simulink model "CubeSatSimulationModel"  (R2024b)
settings: Solver=VariableStepAuto  StartTime=0.0  StopTime=500  MaxStep=0.2  RelTol=1e-3
undefined symbols (not defined in the file or in its folder): IAU, juliandate, mtq, sat, WMM2020
libraries: matrix_library x10, aerolibutil x9, sharedutil x4, aerolibgravity2 x2, simulink_extras x2, sharedtransform x2, aerolibtransform2 x1, simulink x1
settings Model: PacingRate=3  Creator=Ameya  LastModifiedBy=Ameya
settings SFSimCC: SFSimEcho=off
settings RTWCC: GPUComputeCapability=3.5

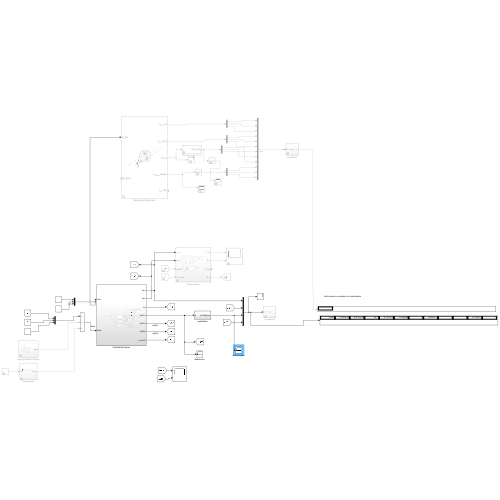
[thumbnail: Simulink's stored preview of the top-level diagram]
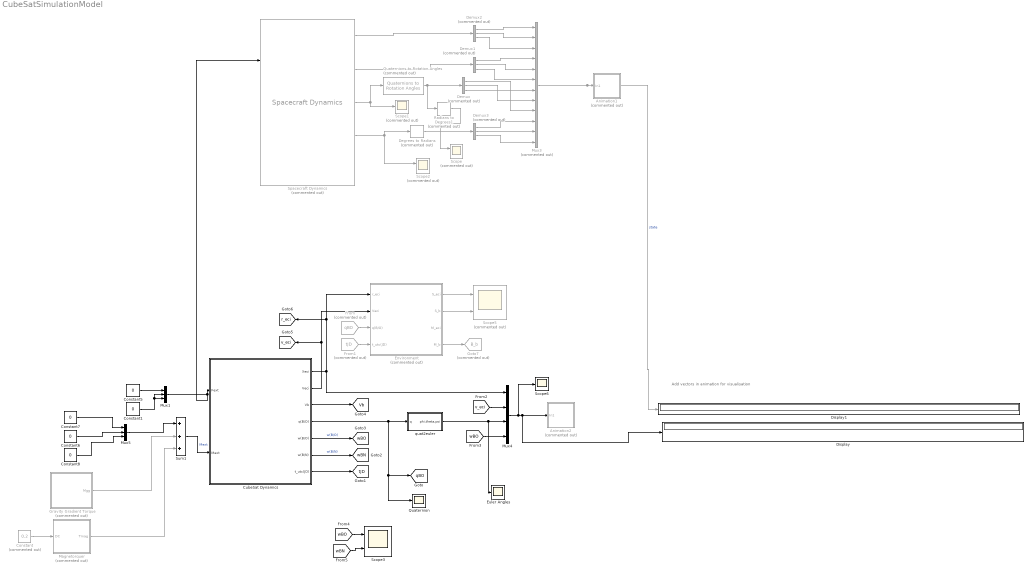
== system CubeSatSimulationModel ==
  note: Add vectors in animation for visualisation
  Animation1 : Subsystem  Commented=on
  Animation2 : Subsystem  Commented=on
  Constant : Constant  Commented=on  Value=0.2
  Constant{1,5..8} (5 alike) : Constant  Value=0
  CubeSat Dynamics : Subsystem
  Degrees to Radians : simulink_extras/Transformations/Degrees to Radians  Commented=on
  Demux{,1..3} (4 alike) : Demux  Commented=on  Outputs=3
  Display : Display
  Display1 : Display
  Environment : Subsystem  Commented=on
  Euler Angles : Scope
  From : From  Commented=on  GotoTag=qBO  TagVisibility=global
  From1 : From  Commented=on  GotoTag=tJD  TagVisibility=global
  Goto7 : Goto  Commented=on  GotoTag=B_b  TagVisibility=global
  Gravity Gradient Torque : Subsystem  Commented=on
  Magnetorquer : Subsystem  Commented=on
  Mux1 : Mux  Inputs=3
  Mux3 : Mux  Commented=on  Inputs=12
  Mux4 : Mux
  Mux5 : Mux  Inputs=3
  Quaternion : Scope
  Quaternions to Rotation Angles : sharedtransform/Quaternions to Rotation Angles  Commented=on  rotationOrder=ZYX  aMode=aMode
  Radians to Degrees1 : simulink_extras/Transformations/Radians to Degrees  Commented=on
  Scope : Scope  Commented=on  NumInputPorts=2
  Scope1 : Scope  Commented=on
  Scope2 : Scope  Commented=on  NumInputPorts=2
  Scope3 : Scope  NumInputPorts=2
  Scope5 : Scope  Commented=on  NumInputPorts=2
  Scope6 : Scope
  Spacecraft Dynamics : SpacecraftDynamics  Commented=on  mass=sat.mass  inertia=sat.J  semiMajorAxis=sat.a  eccentricity=sat.e  inclination=rad2deg(sat.i)  raan=rad2deg(sat.RAAN)  argPeriapsis=rad2deg(sat.w)  trueAnomaly=0  attitudeFrame=LVLH  attitudeRate=rad2deg(sat.w0)
  Sum1 : Sum  Inputs=+++
  quat2euler : Subsystem
  tag scope: Vb=global, qBO=global, r_eci=global, tJD=global, v_eci=global, wBN=global, wBO=global
  wires:
  Spacecraft Dynamics/3 -> Scope1/1, Quaternions to Rotation Angles/1
  Quaternions to Rotation Angles/1 -> Demux/1, Radians to Degrees1/1
  Mux1/1 -> Spacecraft Dynamics/1, CubeSat Dynamics/1(Fext)
  Constant1/1 -> Mux1/2, Mux1/3
  Mux3/1 -> Animation1/1(In1), Display1/1  "state"
  Spacecraft Dynamics/2 -> Demux1/1
  Spacecraft Dynamics/1 -> Demux2/1
  Demux2/1 -> Mux3/1
  Demux2/2 -> Mux3/2
  Demux2/3 -> Mux3/3
  Demux1/1 -> Mux3/4
  Demux1/2 -> Mux3/5
  Demux1/3 -> Mux3/6
  Demux/1 -> Mux3/9
  Demux/2 -> Mux3/8
  Demux/3 -> Mux3/7
  Spacecraft Dynamics/4 -> Scope2/1, Degrees to Radians/1
  Demux3/1 -> Mux3/10
  Demux3/2 -> Mux3/11
  Demux3/3 -> Mux3/12
  Degrees to Radians/1 -> Demux3/1
  Radians to Degrees1/1 -> Scope/1
  CubeSat Dynamics/3(Vb) -> [Vb]
  Mux4/1 -> Scope6/1, Display/1, Animation2/1(In1)
  Constant5/1 -> Mux1/1
  quat2euler/1(phi,theta,psi) -> Mux4/3, Euler Angles/1
  CubeSat Dynamics/6(w(B/N)) -> [wBN]  "w(B/N)"
  CubeSat Dynamics/4(q(B/O)) -> [qBO], Quaternion/1, quat2euler/1(q)
  CubeSat Dynamics/1(Xeci) -> Environment/1(r_eci), [r_eci], Mux4/1
  From1/1 -> Environment/4(t_utc(JD))
  Environment/2(S_b) -> Scope5/2
  CubeSat Dynamics/2(Veci) -> [v_eci], Environment/2(Veci)
  From/1 -> Environment/3(q(B/O))
  CubeSat Dynamics/7(t_utc(JD)) -> [tJD]
  Environment/1(S_eci) -> Scope5/1
  Gravity Gradient Torque/1(Mgg) -> Sum1/2
  Mux5/1 -> Sum1/1
  Constant6/1 -> Mux5/2
  Sum1/1 -> CubeSat Dynamics/2(Mext)  "Mext"
  Constant8/1 -> Mux5/3
  Constant7/1 -> Mux5/1
  CubeSat Dynamics/5(w(B/O)) -> [wBO]  "w(B/O)"
  [v_eci] -> Mux4/2
  [wBO] -> Mux4/4
  Environment/4(M_b) -> Goto7/1
  Magnetorquer/1(Tmag) -> Sum1/3
  Constant/1 -> Magnetorquer/1(DC)
  [wBO] -> Scope3/1
  [wBN] -> Scope3/2

== system CubeSatSimulationModel/Animation1 ==
  In1 : Inport
  Clock : Clock
  CubeSat Attitude Animation : MATLABFcn  MATLABFcn=drawCubeSat  OutputDimensions=0
  Mux1 : Mux  Inputs=2
  wires:
  Mux1/1 -> CubeSat Attitude Animation/1
  In1/1 -> Mux1/1
  Clock/1 -> Mux1/2  "time"

== system CubeSatSimulationModel/Animation2 ==
  In1 : Inport
  Clock : Clock
  CubeSat Attitude Animation : MATLABFcn  MATLABFcn=drawCubeSat  OutputDimensions=0
  Mux1 : Mux  Inputs=2
  wires:
  Mux1/1 -> CubeSat Attitude Animation/1
  In1/1 -> Mux1/1
  Clock/1 -> Mux1/2  "time"

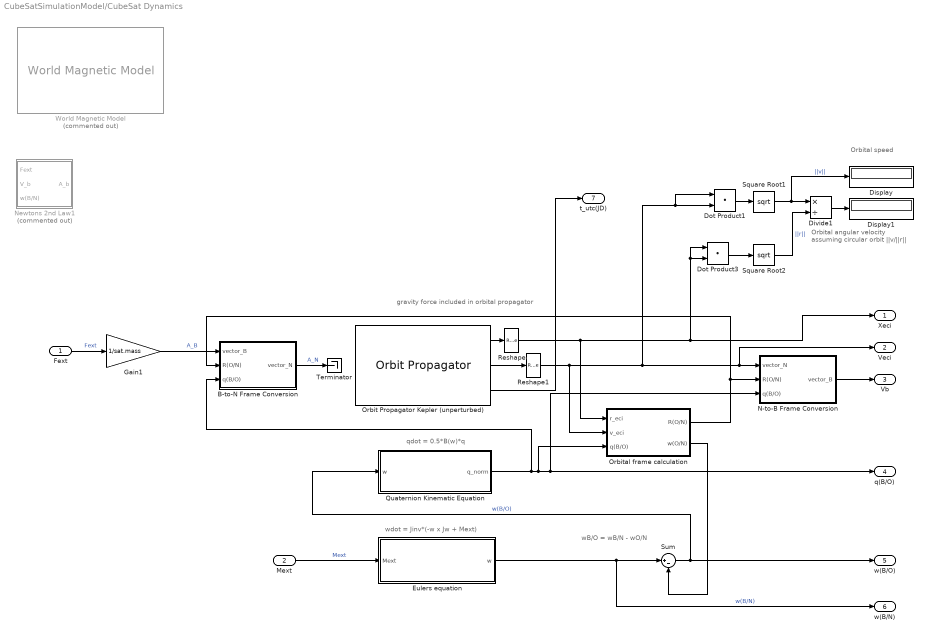
== system CubeSatSimulationModel/CubeSat Dynamics ==
  note: Orbital speed
  note: gravity force included in orbital propagator
  note: Orbital angular velocity
      | assuming circular orbit
      | ||v/||r||
  note: qdot = 0.5*B(w)*q
  note: wdot = Jinv*(-w x Jw + Mext)
  note: wB/O = wB/N - wO/N
  Fext : Inport
  Mext : Inport  Port=2
  B-to-N Frame Conversion : Subsystem
  Display : Display
  Display1 : Display
  Divide1 : Product  Inputs=*/
  Dot Product1 : DotProduct  OutDataTypeStr=Inherit: Inherit via internal rule
  Dot Product3 : DotProduct  OutDataTypeStr=Inherit: Inherit via internal rule
  Eulers equation : Subsystem
  Gain1 : Gain  Gain=1/sat.mass
  N-to-B Frame Conversion : Subsystem
  Newtons 2nd Law1 : Subsystem  Commented=on
  Orbit Propagator Kepler (unperturbed) : OrbitPropagator  accelIn=on  startDate=juliandate(2025, 1, 1, 12, 0, 0)  semiMajorAxis=sat.a  eccentricity=sat.e  inclination=rad2deg(sat.i)  raan=rad2deg(sat.RAAN)  argPeriapsis=rad2deg(sat.w)  trueAnomaly=rad2deg(sat.ta)  inertialPosition=[3649700.0 3308200.0 -4676600.0]  inertialVelocity=[-2750.8 6666.4 2573.4]  fixedPosition=[-4142689.0 -2676864.7 -4669861.6]  fixedVelocity=[1452.7 -6720.7 2568.1]  gravityModel=Oblate ellipsoid (J2)  customR=3396200  customMu=4.305e13  customJ2=1.0826269e-03  customOmega=4.06125949e-3
  Orbital frame calculation : Subsystem
  Quaternion Kinematic Equation : Subsystem
  Reshape : Reshape  OutputDimensionality=Column vector (2-D)
  Reshape1 : Reshape  OutputDimensionality=Column vector (2-D)
  Square Root1 : Sqrt
  Square Root2 : Sqrt
  Sum : Sum  Inputs=|+-
  Terminator : Terminator
  World Magnetic Model : aerolibgravity2/World Magnetic Model  Commented=on  model=WMM2020 (2020-2025)  customFile='WMM2020.COF'  units=Metric (MKS)  time_in=on  month=January  day=1  year=2020  action=Error  h_out=on  dec_out=on  inc_out=on  ti_out=on
  Xeci : Outport
  Veci : Outport  Port=2
  Vb : Outport  Port=3
  q(B/O) : Outport  Port=4
  w(B/O) : Outport  Port=5
  w(B/N) : Outport  Port=6
  t_utc(JD) : Outport  Port=7
  wires:
  Orbit Propagator Kepler (unperturbed)/1 -> Reshape/1
  Orbit Propagator Kepler (unperturbed)/2 -> Reshape1/1
  Reshape1/1 -> Dot Product1/1, Dot Product1/2, Veci/1, N-to-B Frame Conversion/1(vector_N), Orbital frame calculation/2(v_eci)
  Mext/1 -> Eulers equation/1(Mext)  "Mext"
  Eulers equation/1(w) -> w(B/N)/1, Sum/1  "w(B/N)"
  Sum/1 -> Quaternion Kinematic Equation/1(w), w(B/O)/1  "w(B/O)"
  Dot Product1/1 -> Square Root1/1
  Square Root1/1 -> Display/1, Divide1/1  "||v||"
  Dot Product3/1 -> Square Root2/1
  Square Root2/1 -> Divide1/2  "||r||"
  Divide1/1 -> Display1/1
  Quaternion Kinematic Equation/1(q_norm) -> q(B/O)/1, N-to-B Frame Conversion/3(q(B/O)), Orbital frame calculation/3(q(B/O)), B-to-N Frame Conversion/3(q(B/O))
  Orbital frame calculation/2(w(O/N)) -> Sum/2
  Reshape/1 -> Dot Product3/1, Dot Product3/2, Xeci/1, Orbital frame calculation/1(r_eci)
  Orbital frame calculation/1(R(O/N)) -> N-to-B Frame Conversion/2(R(O/N)), B-to-N Frame Conversion/2(R(O/N))
  Fext/1 -> Gain1/1  "Fext"
  N-to-B Frame Conversion/1(vector_B) -> Vb/1
  Gain1/1 -> B-to-N Frame Conversion/1(vector_B)  "A_B"
  B-to-N Frame Conversion/1(vector_N) -> Terminator/1  "A_N"
  Orbit Propagator Kepler (unperturbed)/3 -> t_utc(JD)/1

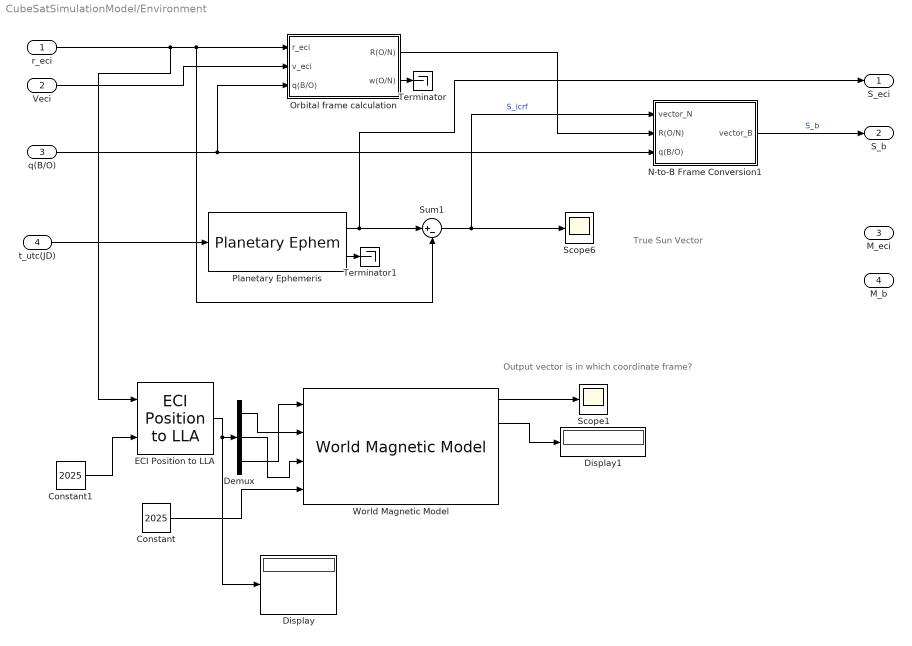
== system CubeSatSimulationModel/Environment ==
  note: Output vector is in which coordinate frame?
  note: True Sun Vector
  r_eci : Inport
  Veci : Inport  Port=2
  q(B/O) : Inport  Port=3
  t_utc(JD) : Inport  Port=4
  Constant : Constant  Value=2025
  Constant1 : Constant  Value=2025
  Demux : Demux  Outputs=3
  Display : Display
  Display1 : Display
  ECI Position to LLA : aerolibtransform2/ECI Position to LLA  red=IAU-2000/2006  year=2025  month=January  day=1  hour=0  min=0  sec=0  deltaT=Day  errorflag=Error  extraparamflag=off  eunits=Metric (MKS)  earthmodel=WGS84  flat=1/298.257223563  eqradius=6378137
      settings: AttributesFormatString=%<red>
  N-to-B Frame Conversion1 : Subsystem
  Orbital frame calculation : Subsystem
  Planetary Ephemeris : PlanetaryEphem  target=Sun
  Scope1 : Scope
  Scope6 : Scope
  Sum1 : Sum  Inputs=|+-
  Terminator : Terminator
  Terminator1 : Terminator
  World Magnetic Model : aerolibgravity2/World Magnetic Model  model=WMM2020 (2020-2025)  customFile='WMM2020.COF'  units=Metric (MKS)  time_in=on  month=January  day=1  year=2020  action=Error  h_out=on  dec_out=on  inc_out=on  ti_out=on
  S_eci : Outport
  S_b : Outport  Port=2
  M_eci : Outport  Port=3
  M_b : Outport  Port=4
  wires:
  Orbital frame calculation/1(R(O/N)) -> N-to-B Frame Conversion1/2(R(O/N))
  Sum1/1 -> Scope6/1, N-to-B Frame Conversion1/1(vector_N)  "S_icrf"
  Planetary Ephemeris/1 -> Sum1/1, S_eci/1
  q(B/O)/1 -> N-to-B Frame Conversion1/3(q(B/O)), Orbital frame calculation/3(q(B/O))
  r_eci/1 -> ECI Position to LLA/1, Orbital frame calculation/1(r_eci), Sum1/2
  t_utc(JD)/1 -> Planetary Ephemeris/1
  N-to-B Frame Conversion1/1(vector_B) -> S_b/1  "S_b"
  Planetary Ephemeris/2 -> Terminator1/1
  Orbital frame calculation/2(w(O/N)) -> Terminator/1
  Veci/1 -> Orbital frame calculation/2(v_eci)
  Demux/3 -> World Magnetic Model/1
  Demux/1 -> World Magnetic Model/2
  Demux/2 -> World Magnetic Model/3
  World Magnetic Model/1 -> Scope1/1
  Constant1/1 -> ECI Position to LLA/2
  Constant/1 -> World Magnetic Model/4
  ECI Position to LLA/1 -> Display/1, Demux/1
  World Magnetic Model/2 -> Display1/1

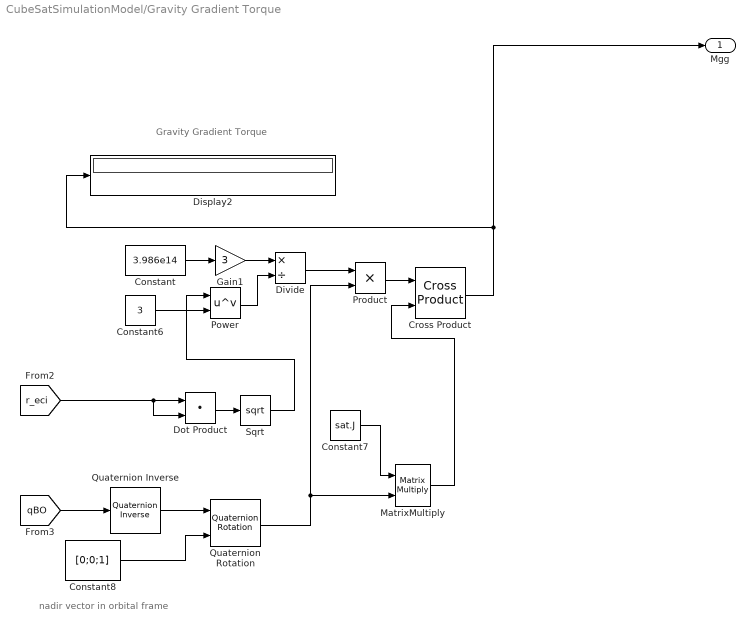
== system CubeSatSimulationModel/Gravity Gradient Torque ==
  note: Gravity Gradient Torque
  note: nadir vector in orbital frame
  Constant : Constant  Value=3.986e14
  Constant6 : Constant  Value=3
  Constant7 : Constant  Value=sat.J
  Constant8 : Constant  Value=[0;0;1]
  Cross Product : matrix_library/Cross Product
  Display2 : Display
  Divide : Product  Inputs=*/
  Dot Product : DotProduct  OutDataTypeStr=Inherit: Inherit via internal rule
  Gain1 : Gain  Gain=3
  MatrixMultiply : Product  Multiplication=Matrix(*)
  Power : Math  Operator=pow
  Product : Product
  Quaternion Inverse : aerolibutil/Quaternion Inverse
  Quaternion Rotation : aerolibutil/Quaternion Rotation
  Sqrt : Sqrt
  Mgg : Outport
  wires:
  Power/1 -> Divide/2
  Cross Product/1 -> Mgg/1, Display2/1
  MatrixMultiply/1 -> Cross Product/2
  Quaternion Inverse/1 -> Quaternion Rotation/1
  [qBO] -> Quaternion Inverse/1
  Sqrt/1 -> Power/1
  [r_eci] -> Dot Product/2, Dot Product/1
  Product/1 -> Cross Product/1
  Constant6/1 -> Power/2
  Dot Product/1 -> Sqrt/1
  Divide/1 -> Product/1
  Quaternion Rotation/1 -> Product/2, MatrixMultiply/2
  Gain1/1 -> Divide/1
  Constant/1 -> Gain1/1
  Constant8/1 -> Quaternion Rotation/2
  Constant7/1 -> MatrixMultiply/1

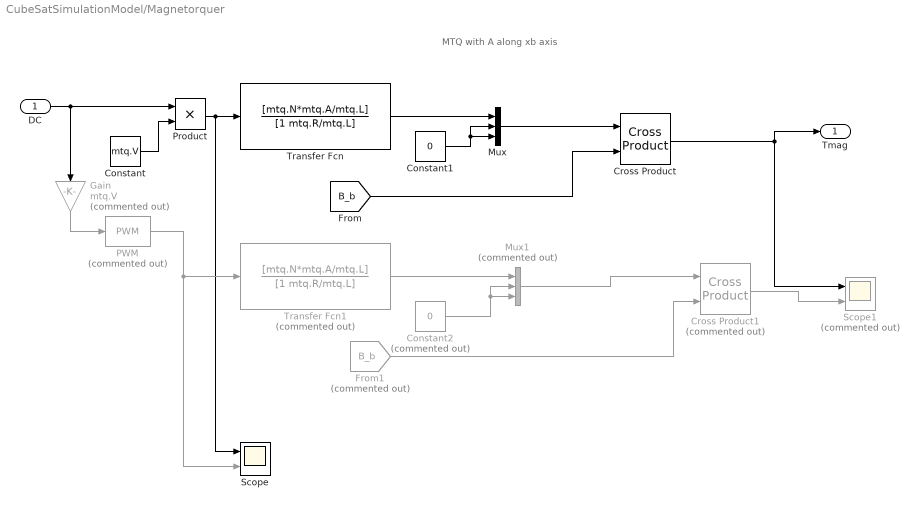
== system CubeSatSimulationModel/Magnetorquer ==
  note: MTQ with A along xb axis
  DC : Inport
  Constant : Constant  Value=mtq.V
  Constant1 : Constant  Value=0
  Constant2 : Constant  Commented=on  Value=0
  Cross Product : matrix_library/Cross Product
  Cross Product1 : matrix_library/Cross Product  Commented=on
  From1 : From  Commented=on  GotoTag=B_b  TagVisibility=global
  Gain : Gain  Commented=on  Gain=mtq.V
  Mux : Mux  Inputs=3
  Mux1 : Mux  Commented=on  Inputs=3
  PWM : simulink/Discontinuities/PWM  Commented=on  DisableCoverage=on  Period=1/50  InitialDelay=0  DisallowZeroDutyCycle=off  RunAtFixedTimeIntervals=off  SampleTime=0.1
  Product : Product
  Scope : Scope  NumInputPorts=2
  Scope1 : Scope  Commented=on  NumInputPorts=2
  Transfer Fcn : TransferFcn  Numerator=[mtq.N*mtq.A/mtq.L]  Denominator=[1 mtq.R/mtq.L]
  Transfer Fcn1 : TransferFcn  Commented=on  Numerator=[mtq.N*mtq.A/mtq.L]  Denominator=[1 mtq.R/mtq.L]
  Tmag : Outport
  wires:
  DC/1 -> Gain/1, Product/1
  Product/1 -> Scope/1, Transfer Fcn/1
  Constant/1 -> Product/2
  Transfer Fcn/1 -> Mux/1
  Cross Product/1 -> Tmag/1, Scope1/1
  [B_b] -> Cross Product/2
  PWM/1 -> Transfer Fcn1/1, Scope/2
  From1/1 -> Cross Product1/2
  Transfer Fcn1/1 -> Mux1/1
  Cross Product1/1 -> Scope1/2
  Constant1/1 -> Mux/2, Mux/3
  Mux/1 -> Cross Product/1
  Constant2/1 -> Mux1/2, Mux1/3
  Mux1/1 -> Cross Product1/1
  Gain/1 -> PWM/1

== system CubeSatSimulationModel/quat2euler ==
  q : Inport
  Demux4 : Demux  Outputs=3
  Mux5 : Mux  Inputs=3
  Quaternions to Rotation Angles1 : sharedtransform/Quaternions to Rotation Angles  rotationOrder=ZYX  aMode=aMode
  phi,theta,psi : Outport
  wires:
  Quaternions to Rotation Angles1/1 -> Demux4/1
  Demux4/3 -> Mux5/1
  Demux4/2 -> Mux5/2
  Demux4/1 -> Mux5/3
  q/1 -> Quaternions to Rotation Angles1/1
  Mux5/1 -> phi,theta,psi/1

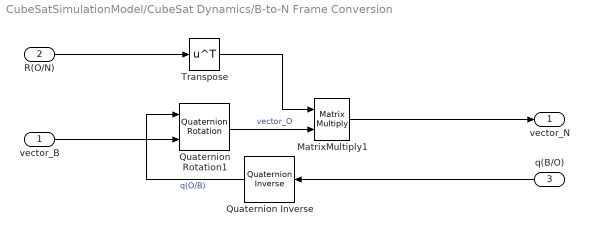
== system CubeSatSimulationModel/CubeSat Dynamics/B-to-N Frame Conversion ==
  vector_B : Inport
  R(O/N) : Inport  Port=2
  q(B/O) : Inport  Port=3
  MatrixMultiply1 : Product  Multiplication=Matrix(*)
  Quaternion Inverse : aerolibutil/Quaternion Inverse
  Quaternion Rotation1 : aerolibutil/Quaternion Rotation
  Transpose : Math  Operator=transpose
  vector_N : Outport
  wires:
  Transpose/1 -> MatrixMultiply1/1
  MatrixMultiply1/1 -> vector_N/1
  R(O/N)/1 -> Transpose/1
  Quaternion Inverse/1 -> Quaternion Rotation1/1  "q(O/B)"
  Quaternion Rotation1/1 -> MatrixMultiply1/2  "vector_O"
  q(B/O)/1 -> Quaternion Inverse/1
  vector_B/1 -> Quaternion Rotation1/2

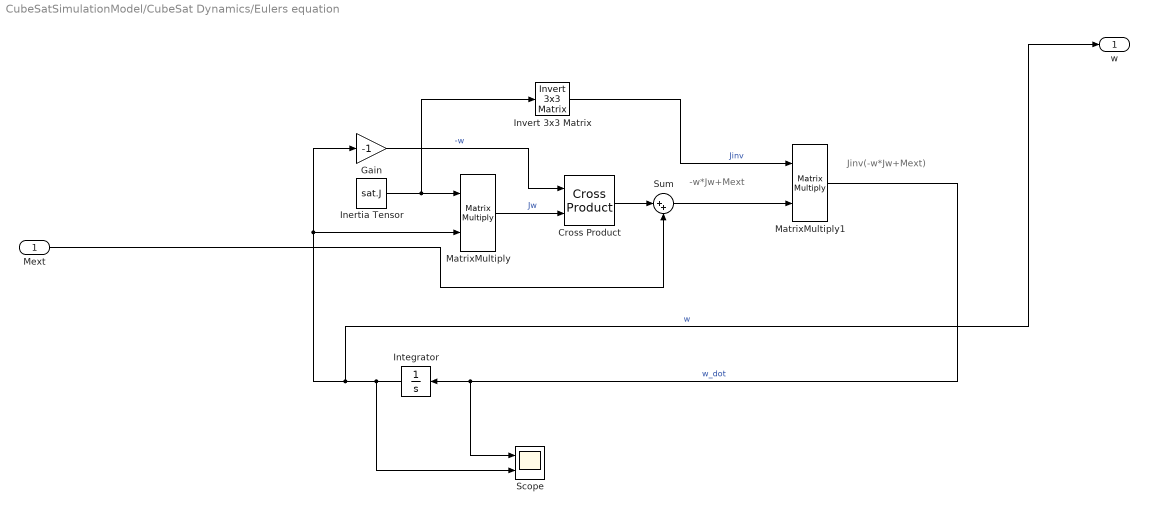
== system CubeSatSimulationModel/CubeSat Dynamics/Eulers equation ==
  note: -w*Jw+Mext
  note: Jinv(-w*Jw+Mext)
  Mext : Inport
  Cross Product : matrix_library/Cross Product
  Gain : Gain  Gain=-1
  Inertia Tensor : Constant  Value=sat.J
  Integrator : Integrator  InitialCondition=sat.omegaBN
  Invert 3x3 Matrix : aerolibutil/Invert  3x3 Matrix
  MatrixMultiply : Product  Multiplication=Matrix(*)
  MatrixMultiply1 : Product  Multiplication=Matrix(*)
  Scope : Scope  NumInputPorts=2
  Sum : Sum  Inputs=|++
  w : Outport
  wires:
  MatrixMultiply/1 -> Cross Product/2  "Jw"
  Invert 3x3 Matrix/1 -> MatrixMultiply1/1  "Jinv"
  MatrixMultiply1/1 -> Scope/1, Integrator/1  "w_dot"
  Inertia Tensor/1 -> Invert 3x3 Matrix/1, MatrixMultiply/1
  Cross Product/1 -> Sum/1
  Sum/1 -> MatrixMultiply1/2
  Gain/1 -> Cross Product/1  "-w"
  Integrator/1 -> Scope/2, w/1, Gain/1, MatrixMultiply/2  "w"
  Mext/1 -> Sum/2

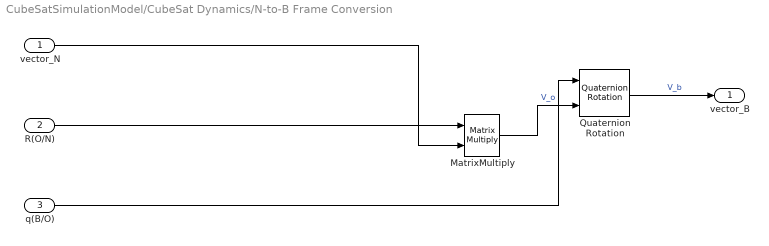
== system CubeSatSimulationModel/CubeSat Dynamics/N-to-B Frame Conversion ==
  vector_N : Inport
  R(O/N) : Inport  Port=2
  q(B/O) : Inport  Port=3
  MatrixMultiply : Product  Multiplication=Matrix(*)
  Quaternion Rotation : aerolibutil/Quaternion Rotation
  vector_B : Outport
  wires:
  MatrixMultiply/1 -> Quaternion Rotation/2  "V_o"
  Quaternion Rotation/1 -> vector_B/1  "V_b"
  R(O/N)/1 -> MatrixMultiply/1
  vector_N/1 -> MatrixMultiply/2
  q(B/O)/1 -> Quaternion Rotation/1

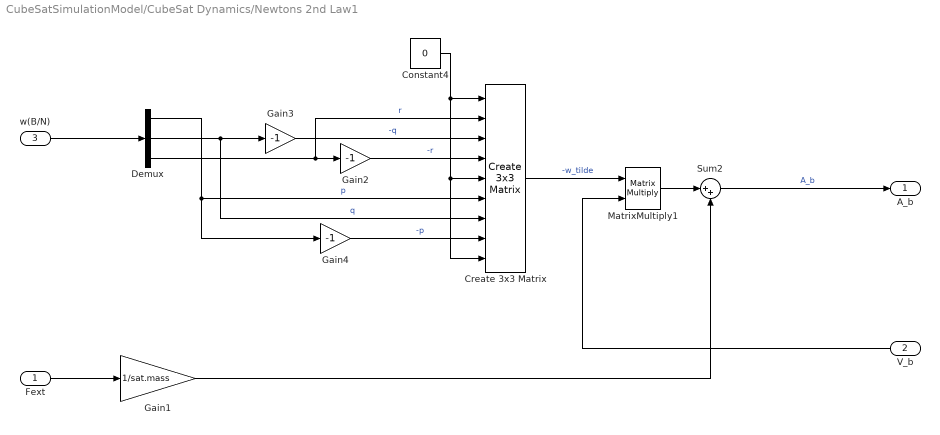
== system CubeSatSimulationModel/CubeSat Dynamics/Newtons 2nd Law1 ==
  Fext : Inport
  V_b : Inport  Port=2
  w(B/N) : Inport  Port=3
  Constant4 : Constant  Value=0
  Create 3x3 Matrix : sharedutil/Create 3x3 Matrix  aMode=aMode
      settings: LibrarySourceBlock=aerolibutil/Create 3x3 Matrix
  Demux : Demux  Outputs=3
  Gain1 : Gain  Gain=1/sat.mass
  Gain2 : Gain  Gain=-1
  Gain3 : Gain  Gain=-1
  Gain4 : Gain  Gain=-1
  MatrixMultiply1 : Product  Multiplication=Matrix(*)
  Sum2 : Sum  Inputs=|++
  A_b : Outport
  wires:
  Constant4/1 -> Create 3x3 Matrix/1, Create 3x3 Matrix/9, Create 3x3 Matrix/5
  Gain2/1 -> Create 3x3 Matrix/4  "-r"
  Fext/1 -> Gain1/1
  Gain4/1 -> Create 3x3 Matrix/8  "-p"
  Demux/2 -> Gain3/1, Create 3x3 Matrix/7  "q"
  Demux/1 -> Create 3x3 Matrix/6, Gain4/1  "p"
  Create 3x3 Matrix/1 -> MatrixMultiply1/1  "-w_tilde"
  Gain1/1 -> Sum2/2
  MatrixMultiply1/1 -> Sum2/1
  Demux/3 -> Create 3x3 Matrix/2, Gain2/1  "r"
  Gain3/1 -> Create 3x3 Matrix/3  "-q"
  V_b/1 -> MatrixMultiply1/2
  Sum2/1 -> A_b/1  "A_b"
  w(B/N)/1 -> Demux/1

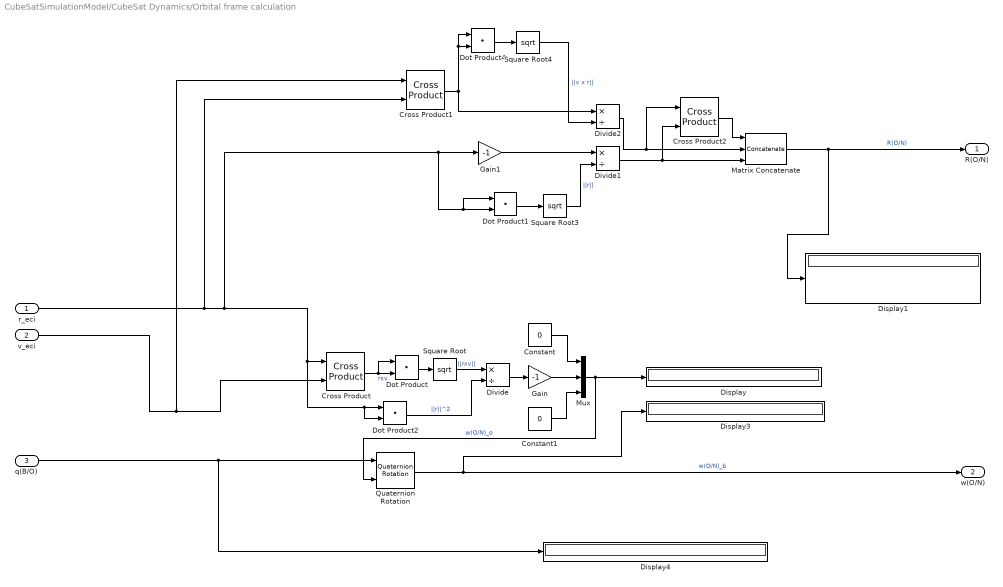
== system CubeSatSimulationModel/CubeSat Dynamics/Orbital frame calculation ==
  r_eci : Inport
  v_eci : Inport  Port=2
  q(B/O) : Inport  Port=3
  Constant : Constant  Value=0
  Constant1 : Constant  Value=0
  Cross Product : matrix_library/Cross Product
  Cross Product1 : matrix_library/Cross Product
  Cross Product2 : matrix_library/Cross Product
  Display{,1,3..4} (4 alike) : Display
  Divide : Product  Inputs=*/
  Divide1 : Product  Inputs=*/
  Divide2 : Product  Inputs=*/
  Dot Product{,1..2,4} (4 alike) : DotProduct  OutDataTypeStr=Inherit: Inherit via internal rule
  Gain : Gain  Gain=-1
  Gain1 : Gain  Gain=-1
  Matrix Concatenate : Concatenate  NumInputs=3  Mode=Multidimensional array  ConcatenateDimension=2
  Mux : Mux  Inputs=3
  Quaternion Rotation : aerolibutil/Quaternion Rotation
  Square Root : Sqrt
  Square Root3 : Sqrt
  Square Root4 : Sqrt
  R(O/N) : Outport
  w(O/N) : Outport  Port=2
  wires:
  Constant1/1 -> Mux/3
  Dot Product2/1 -> Divide/2  "||r||^2"
  Gain/1 -> Mux/2
  q(B/O)/1 -> Quaternion Rotation/1, Display4/1
  Quaternion Rotation/1 -> Display3/1, w(O/N)/1  "w(O/N)_b"
  Cross Product/1 -> Dot Product/1, Dot Product/2  "rxv"
  Dot Product/1 -> Square Root/1
  Divide/1 -> Gain/1
  Square Root/1 -> Divide/1  "||rxv||"
  Mux/1 -> Quaternion Rotation/2, Display/1  "w(O/N)_o"
  Constant/1 -> Mux/1
  Cross Product2/1 -> Matrix Concatenate/1
  Divide2/1 -> Cross Product2/1, Matrix Concatenate/2
  Cross Product1/1 -> Dot Product4/2, Dot Product4/1, Divide2/1
  r_eci/1 -> Cross Product1/2, Dot Product1/1, Dot Product1/2, Gain1/1, Dot Product2/2, Dot Product2/1, Cross Product/1
  Gain1/1 -> Divide1/1
  Square Root3/1 -> Divide1/2  "||r||"
  Square Root4/1 -> Divide2/2  "||v x r||"
  Dot Product1/1 -> Square Root3/1
  v_eci/1 -> Cross Product1/1, Cross Product/2
  Matrix Concatenate/1 -> R(O/N)/1, Display1/1  "R(O/N)"
  Divide1/1 -> Cross Product2/2, Matrix Concatenate/3
  Dot Product4/1 -> Square Root4/1

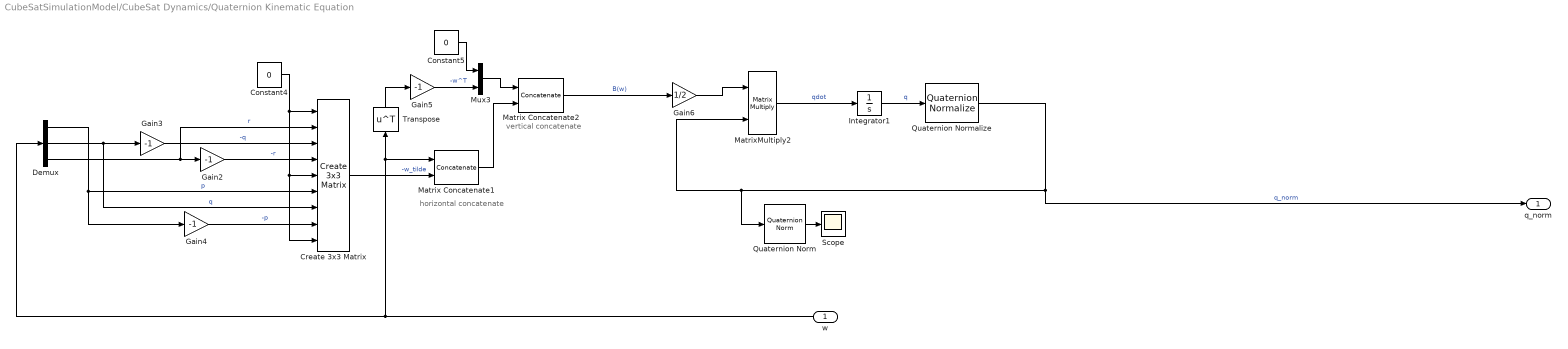
== system CubeSatSimulationModel/CubeSat Dynamics/Quaternion Kinematic Equation ==
  note: horizontal concatenate
  note: vertical concatenate
  w : Inport
  Constant4 : Constant  Value=0
  Constant5 : Constant  Value=0
  Create 3x3 Matrix : sharedutil/Create 3x3 Matrix  aMode=aMode
      settings: LibrarySourceBlock=aerolibutil/Create 3x3 Matrix
  Demux : Demux  Outputs=3
  Gain{2..5} (4 alike) : Gain  Gain=-1
  Gain6 : Gain  Gain=1/2
  Integrator1 : Integrator  InitialCondition=sat.quat
  Matrix Concatenate1 : Concatenate  Mode=Multidimensional array  ConcatenateDimension=2
  Matrix Concatenate2 : Concatenate  Mode=Multidimensional array
  MatrixMultiply2 : Product  Multiplication=Matrix(*)
  Mux3 : Mux  Inputs=2
  Quaternion Norm : sharedutil/Quaternion Norm  aMode=aMode
      settings: LibrarySourceBlock=|
      | aerolibutil/Quaternion
      | Norm
  Quaternion Normalize : sharedutil/Quaternion Normalize  aMode=aMode
  Scope : Scope
  Transpose : Math  Operator=transpose
  q_norm : Outport
  wires:
  Gain5/1 -> Mux3/2  "-w^T"
  Constant4/1 -> Create 3x3 Matrix/1, Create 3x3 Matrix/9, Create 3x3 Matrix/5
  MatrixMultiply2/1 -> Integrator1/1  "qdot"
  Demux/1 -> Create 3x3 Matrix/6, Gain4/1  "p"
  Gain4/1 -> Create 3x3 Matrix/8  "-p"
  Integrator1/1 -> Quaternion Normalize/1  "q"
  Gain2/1 -> Create 3x3 Matrix/4  "-r"
  w/1 -> Demux/1, Transpose/1, Matrix Concatenate1/1
  Mux3/1 -> Matrix Concatenate2/1
  Matrix Concatenate2/1 -> Gain6/1  "B(w)"
  Constant5/1 -> Mux3/1
  Gain6/1 -> MatrixMultiply2/1
  Demux/3 -> Create 3x3 Matrix/2, Gain2/1  "r"
  Gain3/1 -> Create 3x3 Matrix/3  "-q"
  Demux/2 -> Gain3/1, Create 3x3 Matrix/7  "q"
  Quaternion Norm/1 -> Scope/1
  Matrix Concatenate1/1 -> Matrix Concatenate2/2
  Quaternion Normalize/1 -> q_norm/1, Quaternion Norm/1, MatrixMultiply2/2  "q_norm"
  Create 3x3 Matrix/1 -> Matrix Concatenate1/2  "-w_tilde"
  Transpose/1 -> Gain5/1

== system CubeSatSimulationModel/Environment/N-to-B Frame Conversion1 ==
  vector_N : Inport
  R(O/N) : Inport  Port=2
  q(B/O) : Inport  Port=3
  MatrixMultiply : Product  Multiplication=Matrix(*)
  Quaternion Rotation : aerolibutil/Quaternion Rotation
  vector_B : Outport
  wires:
  MatrixMultiply/1 -> Quaternion Rotation/2  "V_o"
  Quaternion Rotation/1 -> vector_B/1  "V_b"
  R(O/N)/1 -> MatrixMultiply/1
  vector_N/1 -> MatrixMultiply/2
  q(B/O)/1 -> Quaternion Rotation/1

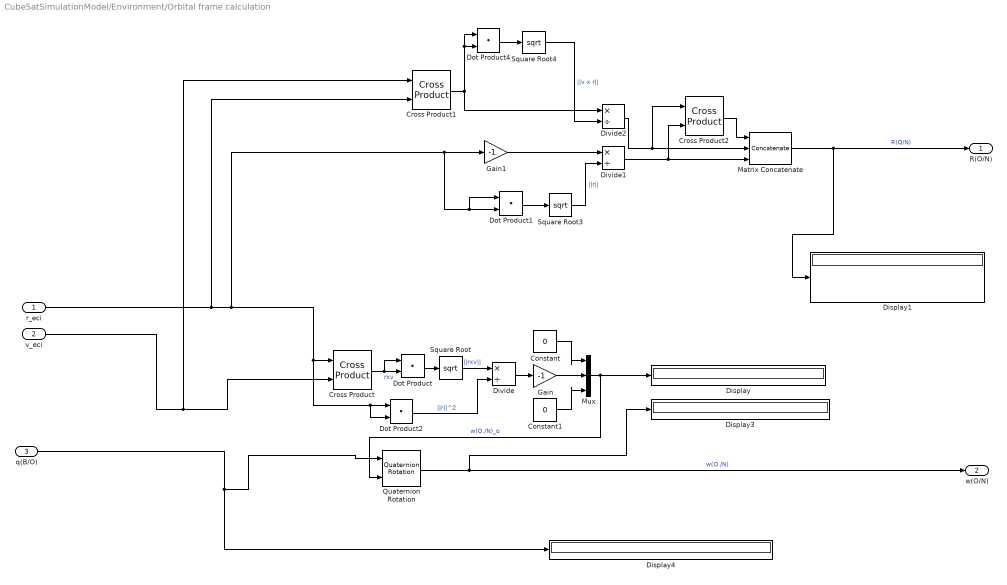
== system CubeSatSimulationModel/Environment/Orbital frame calculation ==
  r_eci : Inport
  v_eci : Inport  Port=2
  q(B/O) : Inport  Port=3
  Constant : Constant  Value=0
  Constant1 : Constant  Value=0
  Cross Product : matrix_library/Cross Product
  Cross Product1 : matrix_library/Cross Product
  Cross Product2 : matrix_library/Cross Product
  Display{,1,3..4} (4 alike) : Display
  Divide : Product  Inputs=*/
  Divide1 : Product  Inputs=*/
  Divide2 : Product  Inputs=*/
  Dot Product{,1..2,4} (4 alike) : DotProduct  OutDataTypeStr=Inherit: Inherit via internal rule
  Gain : Gain  Gain=-1
  Gain1 : Gain  Gain=-1
  Matrix Concatenate : Concatenate  NumInputs=3  Mode=Multidimensional array  ConcatenateDimension=2
  Mux : Mux  Inputs=3
  Quaternion Rotation : aerolibutil/Quaternion Rotation
  Square Root : Sqrt
  Square Root3 : Sqrt
  Square Root4 : Sqrt
  R(O/N) : Outport
  w(O/N) : Outport  Port=2
  wires:
  Constant1/1 -> Mux/3
  Dot Product2/1 -> Divide/2  "||r||^2"
  Gain/1 -> Mux/2
  q(B/O)/1 -> Display4/1, Quaternion Rotation/1
  Quaternion Rotation/1 -> Display3/1, w(O/N)/1  "w(O./N)"
  Cross Product/1 -> Dot Product/1, Dot Product/2  "rxv"
  Dot Product/1 -> Square Root/1
  Divide/1 -> Gain/1
  Square Root/1 -> Divide/1  "||rxv||"
  Mux/1 -> Quaternion Rotation/2, Display/1  "w(O./N)_o"
  Constant/1 -> Mux/1
  Cross Product2/1 -> Matrix Concatenate/1
  Divide2/1 -> Cross Product2/1, Matrix Concatenate/2
  Cross Product1/1 -> Dot Product4/2, Dot Product4/1, Divide2/1
  r_eci/1 -> Cross Product1/2, Dot Product1/1, Dot Product1/2, Gain1/1, Dot Product2/2, Dot Product2/1, Cross Product/1
  Gain1/1 -> Divide1/1
  Square Root3/1 -> Divide1/2  "||r||"
  Square Root4/1 -> Divide2/2  "||v x r||"
  Dot Product1/1 -> Square Root3/1
  v_eci/1 -> Cross Product1/1, Cross Product/2
  Matrix Concatenate/1 -> R(O/N)/1, Display1/1  "R(O/N)"
  Divide1/1 -> Cross Product2/2, Matrix Concatenate/3
  Dot Product4/1 -> Square Root4/1
